simulink model "entrapment_multi"  (R2018a)
settings: Solver=ode23tb  StartTime=0.0  StopTime=Tsim  FixedStep=Tc  RelTol=1e-3
values from neighbouring files (symbols this model uses):
  dsafe = 1    [entrapment.m]
  dsafe_ths = 1    [entrapment.m]
  epsilon_damp = 0.1    [entrapment.m]
  ff = 1 - .5*Tc    (= 0.975)    [entrapment.m]
  k_vo = 1    [entrapment.m]
  l = 2*r*cos(pi/2-pi/n_agents)    [entrapment.m]
  lambda_damp = 0.1    [entrapment.m]
  n_agents = length(q)/2    [compute_centroid.m]    (also in costfun_circular.m; entrapment.m = 9)
  pobs = [ ... (first row only)    [entrapment.m]
  RTPflag = 6    [handle_name.m]    (also in main.m = handle_name(tests(t)))
  starts = zeros(n_agents*2,1)    [entrapment.m]
  Tc = .05    (= 0.05)    [entrapment.m]
  tol = n_agents*r^2/50    (= 18)    [entrapment.m]
settings Model: Creator=anna  LastModifiedBy=anna
settings CodeAppCC: StateflowObjectComments=on

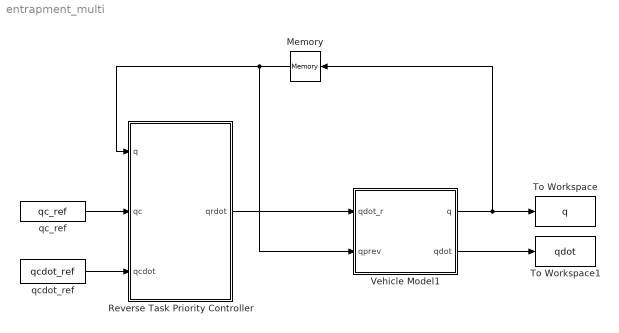
== system entrapment_multi ==
  Memory : Memory  InitialCondition=starts
  Reverse Task Priority Controller : Subsystem
  To Workspace : ToWorkspace  VariableName=q  SaveFormat=Structure With Time  SampleTime=-1
  To Workspace1 : ToWorkspace  VariableName=qdot  SaveFormat=Structure With Time  SampleTime=-1
  Vehicle Model1 : Subsystem  TreatAsAtomicUnit=on
  qc_ref : FromWorkspace  VariableName=qc_ref  SampleTime=Tc
  qcdot_ref : FromWorkspace  VariableName=qcdot_ref  SampleTime=Tc
  wires:
  Vehicle Model1/2(qdot) -> To Workspace1/1
  Vehicle Model1/1(q) -> Memory/1, To Workspace/1
  Reverse Task Priority Controller/1(qrdot) -> Vehicle Model1/1(qdot_r)
  qcdot_ref/1 -> Reverse Task Priority Controller/3("qcdot ")
  qc_ref/1 -> Reverse Task Priority Controller/2(qc)
  Memory/1 -> Vehicle Model1/2(qprev), Reverse Task Priority Controller/1(q)

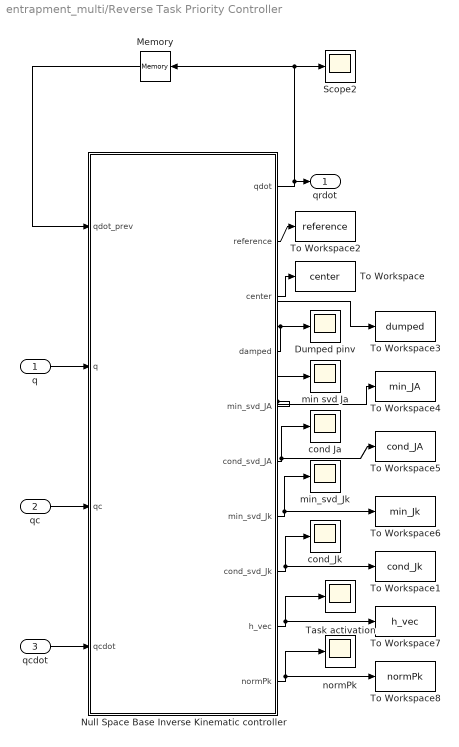
== system entrapment_multi/Reverse Task Priority Controller ==
  q : Inport
  qc : Inport  Port=2
  "qcdot " : Inport  Port=3
  Dumped pinv : Scope
  Memory : Memory  InitialCondition=zeros(2*n_agents,1)  LinearizeMemory=on  LinearizeAsDelay=on
  Null Space Base Inverse Kinematic controller : MATLAB Function  TreatAsAtomicUnit=on
  Scope2 : Scope
  Task activation : Scope
  To Workspace : ToWorkspace  VariableName=center  SampleTime=-1
  To Workspace1 : ToWorkspace  VariableName=cond_Jk  SaveFormat=Structure With Time  SampleTime=-1
  To Workspace2 : ToWorkspace  VariableName=reference  SaveFormat=Structure With Time  SampleTime=-1
  To Workspace3 : ToWorkspace  VariableName=dumped  SaveFormat=Structure With Time  SampleTime=-1
  To Workspace4 : ToWorkspace  VariableName=min_JA  SaveFormat=Structure With Time  SampleTime=-1
  To Workspace5 : ToWorkspace  VariableName=cond_JA  SaveFormat=Structure With Time  SampleTime=-1
  To Workspace6 : ToWorkspace  VariableName=min_Jk  SaveFormat=Structure With Time  SampleTime=-1
  To Workspace7 : ToWorkspace  VariableName=h_vec  SaveFormat=Structure With Time  SampleTime=-1
  To Workspace8 : ToWorkspace  VariableName=normPk  SaveFormat=Structure With Time  SampleTime=-1
  cond Ja : Scope
  cond_Jk : Scope
  min svd Ja : Scope
  min_svd_Jk : Scope
  normPk : Scope
  qrdot : Outport
  wires:
  "qcdot "/1 -> Null Space Base Inverse Kinematic controller/4(qcdot)
  qc/1 -> Null Space Base Inverse Kinematic controller/3(qc)
  q/1 -> Null Space Base Inverse Kinematic controller/2(q)
  Null Space Base Inverse Kinematic controller/7(min_svd_Jk) -> min_svd_Jk/1, To Workspace6/1
  Null Space Base Inverse Kinematic controller/8(cond_svd_Jk) -> cond_Jk/1, To Workspace1/1
  Null Space Base Inverse Kinematic controller/3(center) -> To Workspace/1
  Null Space Base Inverse Kinematic controller/2(reference) -> To Workspace2/1
  Null Space Base Inverse Kinematic controller/1(qdot) -> Memory/1, Scope2/1, qrdot/1
  Null Space Base Inverse Kinematic controller/4(damped) -> To Workspace3/1, Dumped pinv/1
  Null Space Base Inverse Kinematic controller/5(min_svd_JA) -> To Workspace4/1, min svd Ja/1
  Null Space Base Inverse Kinematic controller/6(cond_svd_JA) -> cond Ja/1, To Workspace5/1
  Memory/1 -> Null Space Base Inverse Kinematic controller/1(qdot_prev)
  Null Space Base Inverse Kinematic controller/9(h_vec) -> Task activation/1, To Workspace7/1
  Null Space Base Inverse Kinematic controller/10(normPk) -> normPk/1, To Workspace8/1

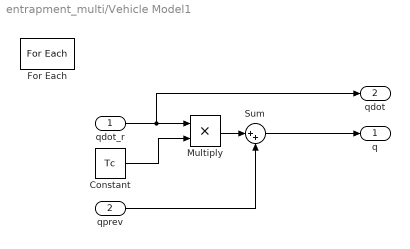
== system entrapment_multi/Vehicle Model1 ==
  qdot_r : Inport  Partition=on  PartitionDimension=1  PartitionWidth=2  PartitionOffset=0
  qprev : Inport  Port=2  Partition=on  PartitionDimension=1  PartitionWidth=2  PartitionOffset=0
  Constant : Constant  Value=Tc
  For Each : ForEach  DisableCoverage=on  IndexMode=One-based
  Multiply : Product
  Sum : Sum  Inputs=|++
  q : Outport  ConcatenationDimension=1
  qdot : Outport  Port=2  ConcatenationDimension=1
  wires:
  qdot_r/1 -> Multiply/1, qdot/1
  qprev/1 -> Sum/2
  Constant/1 -> Multiply/2
  Multiply/1 -> Sum/1
  Sum/1 -> q/1

== matlab function entrapment_multi/Reverse Task Priority Controller/Null Space Base Inverse Kinematic controller ==
  settings: sampleTime=0.05
  data: qdot_prev input; q input; qc input; qcdot input; qdot output; dsafe parameter; dsafe_ths parameter; pobs parameter; reference output; center output; damped output; min_svd_JA output; cond_svd_JA output; RTPflag parameter; min_svd_Jk output; cond_svd_Jk output; l parameter; h_vec output; normPk output; epsilon_damp parameter; k_vo parameter; lambda_damp parameter; ff parameter; tol parameter
function [qdot, reference, center, damped, min_svd_JA, cond_svd_JA, min_svd_Jk, cond_svd_Jk, h_vec, normPk] = NSB_IK_controller(qdot_prev, q, qc, qcdot, dsafe, dsafe_ths, pobs, RTPflag, l, epsilon_damp, k_vo, lambda_damp, ff, tol)
%% Initialization
n_agents = length(q)/2; % 2: (x y) for each agent - hyph. all homogeneous
n_tasks = 2; %number of tasks which may be activated
N = length(q);

% start from a value that is close to the previous computed (low pass
% filtering)
qdot = ff.*qdot_prev; %ATTENTION: if using the gradient, the initial velocity is set differently

% Set this variable according to the total number of subtasks
% which may be activated/deactivated
h_length_ = n_agents*size(pobs,1) + 1; %collision avoidance + centroid

% Damping and svd status (for analysis issues)
damped = zeros(n_tasks+1,1);        % check if the projector has been damped
min_svd_JA = zeros(n_tasks+1,1);	% Lowest singular value of augmented Jacobian
cond_svd_JA = zeros(n_tasks+1,1);	% Condition number of augmented Jacobian
min_svd_Jk = zeros(n_tasks+1,1);
cond_svd_Jk = zeros(n_tasks+1,1);
normPk = zeros(n_tasks+1,1);

coder.extrinsic('weighted_backtr_circ');
coder.extrinsic('costfun_circ');
coder.extrinsic('compute_centroid');
coder.extrinsic('activation_simple');

% used to output the solution and computing tasks and tasks error
reference = zeros(2*n_agents,1); 
center = zeros(2,1);
center = compute_centroid(q);
  
%% Tasks definition

%Task #1: COLLISION AVOIDANCE WITH STATIC OBSTACLE
n_obs = size(pobs,1);
J1 = zeros(n_obs*n_agents,2*n_agents); %preallocation of Jacobians
xdot1 = zeros(n_obs*n_agents,1);       %preallocation of tasks

for j = 1 : n_obs
    for i = 1 : 1 : n_agents
        %Task: distance from the obstacle greater than a threshold
        dcurr = sqrt((q(2*i-1,1)-pobs(j,1))^2 + (q(2*i,1)-pobs(j,2))^2);
        J1((j-1)*n_agents+i,2*i-1:2*i) = (1/dcurr)*[q(2*i-1,1)-pobs(j,1) q(2*i,1)-pobs(j,2)]; %distance between obstacle and robot the goal
        xdot1((j-1)*n_agents+i,1) = .8 * (dsafe+dsafe_ths-dcurr);
    end
end

%Task #6: CENTROID
J6 = zeros(2,2*n_agents);
for i = 1 : n_agents
    J6(:,2*i-1:2*i) = (1/n_agents).*eye(2);                   
end
xdot6 = qcdot(1:2,1) + diag([.8;.8])*(qc(1:2,1)-center);
xdot6 = n_agents*xdot6;
J6 = n_agents*J6;


%Task #9: CIRCULAR
    %Mantaining the formation on a circle without specifying the position
    %of each robot. Both the Jacobians of the paper "Stability
    %analisys ..." are singular when one robot is in the center of the
    %circle and do not ensure to have a task error equal to zero. 
    %Moreover, the value of angle specified in the article is wrong.

J9 = zeros(n_agents,2*n_agents);
xdot9 = zeros(n_agents,1);
r = l/(2*cos(pi/2-pi/n_agents));

pr = zeros(2,1);
%It do not ensure null error even if run without any other task
% for i = 1 : n_agents 
%     pr(1:2) = q(2*i-1:2*i)-qc(1:2);
%     J9(i, 2*i-1:2*i) = pr';
%     xdot9(i) = pr(1:2)'*qcdot(1:2) + .4 * (r^2/2 -.5*(pr(1:2))'*(pr(1:2)));
% end
    for i = 1 : n_agents
        pr(1:2) = q(2*i-1:2*i)-center(1:2, 1);
        for j = 1 : n_agents
            if (j ~= i)
                J9(i, 2*j-1:2*j) = (-1/n_agents).*pr';
            else
                J9(i, 2*j-1:2*j) = (1-1/n_agents).*pr';
            end
        end
        xdot9(i) = .8 * (r^2/2 -.5*(pr(1:2))'*(pr(1:2)));
    end
%This task is singular whenever one of agents poses is equal to the center.
%In this case, the Jacoian is not full rank row and damped pseudoinverse should be used. 

% ATTENTION: Enable this part of the code whether using the gradient to
% initialize the solution (see Section IV.C)
% of the paper "On Null Space-Based Inverse Kinematics Techniques for Fleet
% Management: Toward Time-Varying Task Activation"

% [fun,gradf] = costfun_circular(r,q);
% alpha = 1;  %to let Simulink know the size of the returned argument
% alpha = weighted_backtr_circ(1,q,r);
% if (fun > tol)
%     qdot = -alpha*gradf/norm(gradf);
% else
%     qdot = zeros(size(qdot_prev));
% end

%Task #10: PERIMETER
J10 = zeros(1,2*n_agents);
task_value = .5*(q(1:2)-q(2*(n_agents-1)+1:2*(n_agents-1)+2))'*(q(1:2)-q(2*(n_agents-1)+1:2*(n_agents-1)+2));
for i = 1 : n_agents
    if i > 1 && i < n_agents
        J10(1,2*i-1:2*i) = (q(2*i-1:2*i)-q(2*(i-2)+1:2*(i-1)))'+(q(2*i-1:2*i)-q(2*i+1:2*i+2))';
    else
        if (i == 1)
            J10(1,2*i-1:2*i) = (q(2*i-1:2*i)-q(2*(n_agents-1)+1:2*(n_agents-1)+2))'+(q(2*i-1:2*i)-q(2*i+1:2*i+2))';
        else
            J10(1,2*i-1:2*i) = (q(2*i-1:2*i)-q(2*(i-2)+1:2*(i-1)))'+(q(2*i-1:2*i)-q(1:2))';
        end
    end
    if (i < n_agents)
        task_value = task_value + .5*(q(2*i-1:2*i)-q(2*i+1:2*i+2))'*(q(2*i-1:2*i)-q(2*i+1:2*i+2));
    end
end
xdot10 = .5 * (.5*n_agents*l^2 - task_value);

%% Initializing the stack

J = [];          %stack of Jacobians
coder.varsize('J');

rows = [];          %stack of Jacobians
coder.varsize('rows');

xdot = [];          %stack of Jacobians
coder.varsize('xdot');

%Vector collecting tasks activation for each agent
h_vec = zeros(h_length_+1,1);

% Piling up the task jacobians.
% WARNING: J, xdot, rows and h are ordered buffers. 
%           The first is the task with the highest priority, the last is
%           the task with the lowest priority.
if (RTPflag == 2) %iCAT TCP
    %Adding one more task to saturate the residual degrees of freedom
    %(see the paper )
    n_tasks = n_tasks + 1;
    h_length_ = h_length_ + 1;
    
    %Collision avoidance + centroid
    J = [J1;J6;eye(N)];
    xdot = [xdot1;xdot6;qdot];
    rows = [size(J1,1);size(J6,1);N];
    
    %Centroid + circular + perimeter
%     J = [J6;J9;J10;eye(N)];
%     xdot = [xdot6;xdot9;xdot10;qdot];
%     rows = [size(J6,1);size(J9,1);size(J10,1);N];

    %Collision avoidance + centroid + perimeter (+ gradient to be enabled)
%     J = [J1;J6;J10;eye(N)];
%     xdot = [xdot1;xdot6;xdot10;qdot];
%     rows = [size(J1,1);size(J6,1);size(J10,1);N];

    %Collision avoidance + centroid + circular + perimeter
%     J = [J1;J6;J9;J10;eye(N)];
%     xdot = [xdot1;xdot6;xdot9;xdot10;qdot];
%     rows = [size(J1,1);size(J6,1);size(J9,1);size(J10,1);N];

    rowJ = size(J,1);
else
%    Do similarly
     J = [J1;J6];
     xdot = [xdot1;xdot6];
     rows = [size(J1,1);size(J6,1)];
     rowJ = size(J,1);
end

circular_index = 5; %FIXME not used
collision_avoidance_index = 1; %FIXME not used
        
stack = 0;          % current stack position index

JA_k = [];          % stack of Jacobians
coder.varsize('JA_k');

Jinv = [];          % current Jacobian pseudo-inverse
coder.varsize('Jinv');

Jk = [];            % current Jacobian
coder.varsize('Jk');

H = [];           % Jacobian of current active tasts
coder.varsize('H');

xdotk = [];         % current task value (iteration)
coder.varsize('xdotk');

Hbuff = [];
coder.varsize('Hbuff'); % Buffer storing all the activation matrices

% pre initialize projectors
PAinv = eye(N);
Ptilda = eye(N);

%% Compute qdot according to the method chosen. Check the handle_name function.
if RTPflag == 4 || RTPflag == 2 % 4 is ST, 2 is iCAT-TCP: TOP DOWN TASK PRIORITY ORDERING
    h_index = 0; % start stacking from the higher priority task
    
    %start from a value that is close to the previous computed (low pass
    %filtering)

    %% go through each task
    for i = 1 : n_tasks       
        dq = zeros(N,1);

        % get current task variables
        Jk = J(stack+1:stack+rows(i),:);
        xdotk = xdot(stack+1:stack+rows(i),:);
        
        %% compute activation matrix H (called A in the paper) for each task
        % initializing activation matrix and Jacobians as for bilateral
        % tasks (always active)
        H = eye(size(Jk,1));

        % check activation for unilateral constraints:
        % stack just the not inactive components
        if ( i == collision_avoidance_index )
            
            H = zeros(size(Jk,1)); % clear activation (needs to be recomputed)
            
            % collision avoidance
            counter = 0;
            for k = 1 : size(pobs,1)
                for j = 1 : 1 : n_agents
                    dcurr = sqrt((q(2*j-1,1)-pobs(k,1))^2 + (q(2*j,1)-pobs(k,2))^2);
                    h_index = h_index + 1;
                    counter = counter + 1;
                    h_vec(h_index) = activation_simple('>', dcurr, dsafe, dsafe_ths);
                    H(counter,counter) = h_vec(h_index);
                end
            end
        else
            h_index = h_index + 1;
            h_vec(h_index) = 1;
        end
        
        Hbuff = blkdiag(Hbuff, H);  % collect activation matrices
        JA_k = [JA_k; Jk];          % augmented jacobian
        % %%%%% just for visualization purposes
        s = svd(JA_k);
        min_svd_JA(i) = min(s);
        cond_svd_JA(i) = min_svd_JA(i)/max(s);
        % %%%%%
        %% check if any task is active and process it
        if ( trace(H) > 0 ) % something is active, let's update ...
            
            ind = find(diag(H) > 0);    % collect indices of task active rows
            % %%%% just for visualization purposes
            s = svd(Jk(ind,:));
            min_svd_Jk(i) = rank(Jk(ind,:));%min(s);
            cond_svd_Jk(i) = min_svd_Jk(i)/max(s);
            % %%%%
            
            switch RTPflag   
                case 4 % Standard Approach
                    [JkPAinv, damped(i)] = damped_pinv(Jk(ind,:)*PAinv, lambda_damp, epsilon_damp);
                    normPk(i) = norm(JkPAinv);

                    % compute task contribution
                    dq = PAinv*JkPAinv*H(ind,ind)*(xdotk(ind)-Jk(ind,:)*qdot);

                    % update projector (without damping)               
                    PAinv = PAinv*(eye(N)-JkPAinv*Jk(ind,:)*PAinv);
                    
                    % update projector (with damping)
%                     JkPAinvJkPA = zeros(N);
%                     [u,~,~] = svd(JkPAinv);
%                     for j = 1 : rank(JkPAinv)
%                         JkPAinvJkPA = JkPAinvJkPA + u(:,j)*u(:,j)';
%                     end
%                     PAinv = PAinv*(eye(N) - JkPAinvJkPA);
                
                case 2 % iCAT-TCP
                    epsilon_damp = .1; lambda_damp = .1;
                    [JkPAinv, damped(i), ~] = pinvSC(Jk*PAinv, H, eye(N), 0, epsilon_damp, lambda_damp);
                    [M,d,~] = pinvSC(Jk*PAinv, H, PAinv, k_vo, epsilon_damp, lambda_damp);
                    damped(i) = bitshift(double(damped(i)),1) + d;
                    Wk = Jk*PAinv*M;
                    normPk(i) = norm(PAinv*JkPAinv*Wk);
                    
                    % compute task contribution
                    dq = PAinv*JkPAinv*Wk*(xdotk-Jk*qdot);
                                      
                    % update the projector
                    PAinv = PAinv*(eye(N)-JkPAinv*Jk*PAinv);
            end
            
            %Update
            qdot = qdot + dq;
        end
        stack = stack + rows(i);
    end    
else
    h_index = h_length_ + 1; %stack from the bottom to the top  
    
    for i = n_tasks:-1:1 %Reverse order: from the BOTTOM to the TOP
        
        dq = zeros(N,1);

        %get current task variables
        Jk = J(rowJ-stack-rows(i)+1:rowJ-stack,:);
        xdotk = xdot(rowJ-stack-rows(i)+1:rowJ-stack,:);

        H = eye(size(Jk,1)); % preinitialization as if the task will be bilateral

        %check activation for unilateral constraints
        if ( i == collision_avoidance_index )
            
            H = zeros(size(Jk,1)); % clear activation (needs to be recomputed)
            
            %collision avoidance
            counter = 0;
            for k = 1 : size(pobs,1)
                for j = 1 : 1 : n_agents
                    dcurr = sqrt((q(2*j-1,1)-pobs(k,1))^2 + (q(2*j,1)-pobs(k,2))^2);
                    counter = counter + 1;
                    h_index = h_index - 1;
                    h_vec(h_index) = activation_simple('>', dcurr, dsafe, dsafe_ths);
                    H(counter,counter) = h_vec(h_index);
                end
            end          
        else
            h_index = h_index - 1;
            h_vec(h_index) = 1;
        end
        
        JA_k = [Jk;JA_k];
        Hbuff = blkdiag(H,Hbuff);
        
        s = svd(JA_k);
        min_svd_JA(i) = min(s);
        cond_svd_JA(i) = min_svd_JA(i)/max(s);
                
        if (trace(H) > 0) % something is active, let's update ...
            
            ind = find(diag(H) > 0);
            indbuff = find(diag(Hbuff) > 0);
            
            s = svd(Jk(ind,:));
            min_svd_Jk(i) = rank(Jk(ind,:));%min(s);
            cond_svd_Jk(i) = min_svd_Jk(i)/max(s);

            switch RTPflag
                case 0 %Singularity Robust

                    % Use damping with singular tasks only
                    % connectivity, sphere, variance, circular
                    if ( i == circular_index || i == collision_avoidance_index )
                        [Jkinv, damped(i)] = damped_pinv(Jk(ind,:), lambda_damp, epsilon_damp);
                    else
                        Jkinv = pinv(Jk(ind,:));
                        damped(i) = 0;
                    end

                    % compute task contribution                    
                    innov = H(ind,ind)*(xdotk(ind) - Jk(ind,:)*qdot);
                    dq = Jkinv*innov;
                    normPk(i) = norm(Jkinv*H(ind,ind));

                case 1 %Reverse Priority
                                        
                    %compute Tk matrices (rank-update)
                    [JAinv, damped(i)] = damped_pinv(JA_k(indbuff,:), lambda_damp, epsilon_damp);
                    Tk = JAinv(:,1:length(ind));
                    
                    %%%%%%%%%%%%%%%%% Damped projector
%                     [JkTkpinv, d] = damped_pinv(Jk(ind,:)*Tk, lambda_damp, epsilon_damp);            
%                     damped(i) = bitshift(double(damped(i)),1) + d;
% 
%                     % compute task contribution
%                     innov = H*(xdotk-Jk*qdot);
%                     dq = Tk*JkTkpinv*innov(ind,:);
%                     normPk(i) = norm(Tk*JkTkpinv);
                    
                    %%%%%%%%%%%%%%%%%%
                    
                    % Compute null space and projector (correct in spite of
                    % damping)
                    TkTkinv = zeros(size(Tk,1));
                    [u,~,~] = svd(Tk);
                    for j = 1 : rank(Tk)
                        TkTkinv = TkTkinv + u(:,j)*u(:,j)';
                    end
%                     Tk = orth(JAinv(:,1:length(ind)));
%                     TkTkinv = Tk*pinv(Tk);
                                       
                    JkTkTkinv = Jk(ind,:)*TkTkinv;
                    [JkTkpinv, d] = damped_pinv(JkTkTkinv, lambda_damp, epsilon_damp);            
                    damped(i) = bitshift(double(damped(i)),1) + d;

                    % compute task contribution
                    innov = H*(xdotk-Jk*qdot);
                    dq = JkTkpinv*innov(ind,:);
                    normPk(i) = norm(JkTkpinv);

                case 3 % iCAT-RP
%%%%%%%%%%%%%%%%%%%%%%%%%%%%%%%%%%%%%%%%%%%%%%
                    % compute Tk matrices
                    [JAinv, damped(i),normPk(i)] = pinvSC(JA_k(indbuff,:), Hbuff(indbuff,indbuff), eye(N), 0, epsilon_damp, lambda_damp); %considerando la pseudo-inversa binaria ho maggiore discontinuità
                    Jinv = JAinv*pinv(Hbuff(indbuff,indbuff));
                    Tk = orth(Jinv(:,1:size(Jk(ind),1)));
                    TkTkinv = Tk*pinv(Tk);
%                     Tk = Jinv(:,1:size(Jk,1));
% 
%                     % Compute null space and projector
%                     TkTkinv = zeros(size(Tk,1));
%                     [u,~,~] = svd(Tk);
%                     for j = 1 : rank(Tk)
%                         TkTkinv = TkTkinv + u(:,j)*u(:,j)';
%                     end
                    
                    % Compute null space
                    JAJAinv = JAinv*JA_k(indbuff,:);

                    % compute the continuous projector in the null space of the linearly independent rows 
                    Ptilda = (eye(N)-TkTkinv)*(eye(N)-JAJAinv) + TkTkinv;
%%%%%%%%%%%%%%%%%%%%%%%%%%%%%%%%%%%%%%%%%%%
%                     [JAinv, damped(i),normPk(i)] = pinvSC(JA_k, Hbin, eye(N), 0, epsilon_damp, lambda_damp); %considerando la pseudo-inversa binaria ho maggiore discontinuità
%                     Tk = orth(JAinv(:,1:size(Jk,1)));
%                     TkTkinv = Tk*pinv(Tk);
%                     Ptilda = (eye(N)-TkTkinv)*(eye(N)-JAinv*JA_k) + TkTkinv;

                    % continuous pseudoinversion of JkPtilda, shaped
                    % with the current activation values H
                    [JkTkpinv, d, normPk(i)] = pinvSC(Jk(ind,:)*Ptilda, H(ind,ind), eye(N), 0, epsilon_damp, lambda_damp);
                    damped(i) = bitshift(double(damped(i)),1) + d;

                    % update the law
                    dq = Ptilda*JkTkpinv*(xdotk(ind)-Jk(ind,:)*qdot); %already contains the H
                    %normPk(i) = norm(Ptilda*JkTkpinv);
                      

                case 5 %iCAT-SR
                    epsilon_damp = .1; lambda_damp = .1;
                    [Jkinv, damped(i)] = pinvSC(Jk, H, eye(N), 0, epsilon_damp, lambda_damp);
                    dq = Jkinv*(xdotk-Jk*qdot);  
                    normPk(i) = norm(Jkinv);
                    
                case 6 %Conservative iCAT-RP
                    
                    %compute Tk matrices using pinvSC just with the SVO
                    %component active (just setting the activation matrix
                    %to be equal to the identity you are disabling the task
                    %oriented component).
                    [JAinv, damped(i)] = pinvSC(JA_k, eye(size(JA_k,1)), eye(N), 0, epsilon_damp, lambda_damp); %è la pseudoinversa classica
                    Tk = JAinv(:,1:size(Jk,1));

                    %Compute null space and projector
                    TkTkinv = zeros(size(Tk,1));
                    [u,~,~] = svd(Tk);
                    for j = 1 : rank(Tk)
                        TkTkinv = TkTkinv + u(:,j)*u(:,j)';
                    end
                    
                    %iterative law to speed up the computation (if tk
                    %computed as rank update)
                    Ptilda = (eye(N)-TkTkinv)*PAinv+TkTkinv;
                    PAinv = (eye(N)-Tk*Jk)*PAinv+Tk*(eye(size(H,1))-H)*Jk;

                    %compute the continuous pseudoinverse
                    [JkTkpinv, d, ~] = pinvSC(Jk*Ptilda, H, eye(N), 0, epsilon_damp, lambda_damp);
                    damped(i) = bitshift(double(damped(i)),1) + d;

                    dq = Ptilda*JkTkpinv*(xdotk-Jk*qdot);
                    normPk(i) = norm(eye(N)-TkTkinv);%norm((eye(N)-TkTkinv)*PAinv);
            end

            %Update
            qdot = qdot + dq;
        end                    

        %increment index
        stack = stack + rows(i);
    end
end
